simulink model "ConfiguredVirtualVehicleModel"  (R2023b)
settings: configuration reference "VehicleVariable" (kept outside this file)
StartFcn:
  | %tic
StopFcn:
  | %toc
model workspace (MAT data in the model file):
  ExtDrvCmdsSwitch : Simulink.Parameter (value not decoded)
  ExtDrvRefSwitch : Simulink.Parameter (value not decoded)
  ExtEnvSwitch : Simulink.Parameter (value not decoded)
  ExtGndSwitch : Simulink.Parameter (value not decoded)
values from neighbouring files (symbols this model uses):
  L = 2.79    [EVFmincon_custom.m]
symbols that are objects in the model workspace (value not decoded): ExtDrvCmdsSwitch, ExtDrvRefSwitch, ExtEnvSwitch, ExtGndSwitch
undefined symbols (not defined in the file or in its folder): AccelCmd, AmbTemp, BaroPress, CtrlTcuInitGear, CtrlVcuCltch1InitCmd, CurvGradRef, CurvRef, DCM, DecelCmd, Disabled, DriverAeroRes, DriverDrivelineRes, DriverInitialGear, DriverPreviewDist, DriverRollRes, DriverShiftTime, DriverTimeConst, DriverTractiveForce, EnvAbsPrs, EnvAirTemp, EnvGrvty, EnvNomFrictionScaling, EnvNominalGrade, EnvWindVelX, EnvWindVelY, EnvWindVelZ, FTP75, Gnd, Grade, HazzardCmd, HighBeamCmd, lambda_mux, LeftSignalCmd, LngRef, LowBeamCmd, LtrRef, PhiRef, PlntVehDstCGFrntAxl, PlntVehDstCGRearAxl, PlntVehInitLatPos, PlntVehInitLongPos, PlntVehInitPitchAng, PlntVehInitRollAng, PlntVehInitVertPos, PlntVehInitYawAng, PlntVehMass, PlntVehTrckWdth, PlntVehYawMomentInertia, PlntWhlLdRadius, RightSignalCmd, ScnCRMaxLatAccel, ScnCRRadius, ScnDLCGateLongPos, ScnDLCLatRef, ScnDLCLatRefOffset, ScnDLCLongRefBpt, ScnDLCLongRefStartPos, ScnDLCVehicleWidth, ScnFHCounterDwellTime, ScnFHInitialDwellTime ... (+22)
libraries: simulink x27, autolibutils x8, vehdynlibscenariocommon x7, vehdynlibviscommon x3, vehdynlibdriver x2, sim3dgroundtruthsensorlib x2, autolibshared x2, vrlib x1, autolibsharedcommon x1, sharedtransform x1, sim3dlib x1, sim3dautolib x1
(part 5 of 6)

== system ConfiguredVirtualVehicleModel/Driver Commands/Driver Commands/Longitudinal Driver/Hill Hold & Stop/Hill Hold ==
  <EngSpdOut> : Inport
  <xdot> : Inport  Port=2
  <BattSoc> : Inport  Port=3
  LngRef : Inport  Port=4
  <Grade> : Inport  Port=5
  Abs : Abs  ZeroCross=off  SaturateOnIntegerOverflow=off
  Abs1 : Abs  ZeroCross=off  SaturateOnIntegerOverflow=off
  Compare To Constant : simulink/Logic and Bit Operations/Compare To Constant  relop=<=  const=.1  OutDataTypeStr=boolean  ZeroCross=off
  Compare To Constant1 : simulink/Logic and Bit Operations/Compare To Constant  relop=>=  const=.1  OutDataTypeStr=boolean  ZeroCross=off
  Compare To Constant2 : simulink/Logic and Bit Operations/Compare To Constant  relop=<=  const=500  OutDataTypeStr=boolean  ZeroCross=off
  Compare To Constant3 : simulink/Logic and Bit Operations/Compare To Constant  relop=<=  const=5  OutDataTypeStr=boolean  ZeroCross=off
  Compare To Constant4 : simulink/Logic and Bit Operations/Compare To Constant  relop=<=  const=.1  OutDataTypeStr=boolean  ZeroCross=off
  Data Type Conversion1 : DataTypeConversion  SaturateOnIntegerOverflow=off  RndMeth=Floor
  Logical Operator : Logic  AllPortsSameDT=off  OutDataTypeStr=boolean
  Logical Operator1 : Logic  Inputs=3  AllPortsSameDT=off  OutDataTypeStr=boolean
  Logical Operator2 : Logic  Operator=OR  AllPortsSameDT=off  OutDataTypeStr=boolean
  Signal Specification : SignalSpecification  Unit=m/s
  Unit Conversion : UnitConversion
  DecelOvr : Outport
  EnblDecelOvr : Outport  Port=2
  wires:
  Compare To Constant/1 -> Logical Operator/1
  Unit Conversion/1 -> Signal Specification/1
  Logical Operator2/1 -> DecelOvr/1, Data Type Conversion1/1
  Abs1/1 -> Compare To Constant1/1
  LngRef/1 -> Abs/1
  Compare To Constant1/1 -> Logical Operator/2
  Compare To Constant3/1 -> Logical Operator1/2
  Logical Operator/1 -> Logical Operator2/2
  Compare To Constant2/1 -> Logical Operator1/1
  Data Type Conversion1/1 -> EnblDecelOvr/1
  Logical Operator1/1 -> Logical Operator2/1
  Abs/1 -> Compare To Constant/1
  Signal Specification/1 -> Compare To Constant3/1
  <EngSpdOut>/1 -> Compare To Constant2/1
  Compare To Constant4/1 -> Logical Operator1/3
  <Grade>/1 -> Abs1/1
  <xdot>/1 -> Unit Conversion/1
  <BattSoc>/1 -> Compare To Constant4/1

== system ConfiguredVirtualVehicleModel/Driver Commands/Driver Commands/Longitudinal Driver/Hill Hold & Stop/Stop Detection ==
  LngRef : Inport
  <xdot> : Inport  Port=2
  Abs2 : Abs  ZeroCross=off  SaturateOnIntegerOverflow=off
  Compare To Constant5 : simulink/Logic and Bit Operations/Compare To Constant  relop=<=  const=.1  OutDataTypeStr=boolean  ZeroCross=off
  Compare To Constant6 : simulink/Logic and Bit Operations/Compare To Constant  relop===  const=0  OutDataTypeStr=boolean  ZeroCross=off
  Cont LPF : autolibutils/Cont LPF  wc=2*pi*40  AbsoluteTolerance=auto  aMode=6
  Data Type Conversion2 : DataTypeConversion  SaturateOnIntegerOverflow=off  RndMeth=Floor
  Gain : Gain  Gain=.1
  LatchSwitchCont : autolibutils/LatchSwitchCont  aMode=6
  Logical Operator1 : Logic  Operator=NOT  AllPortsSameDT=off  OutDataTypeStr=boolean
  Logical Operator3 : Logic  AllPortsSameDT=off  OutDataTypeStr=boolean
  DecelOvrCmd : Outport
  EnblDecelOvr : Outport  Port=2
  wires:
  Compare To Constant5/1 -> Logical Operator3/1
  Logical Operator3/1 -> LatchSwitchCont/1
  LngRef/1 -> Compare To Constant6/1
  Abs2/1 -> Compare To Constant5/1
  LatchSwitchCont/1 -> EnblDecelOvr/1, Data Type Conversion2/1
  Data Type Conversion2/1 -> Gain/1
  Logical Operator1/1 -> LatchSwitchCont/2
  Compare To Constant6/1 -> Logical Operator1/1, Logical Operator3/2
  Gain/1 -> Cont LPF/1
  Cont LPF/1 -> DecelOvrCmd/1
  <xdot>/1 -> Abs2/1

== system ConfiguredVirtualVehicleModel/Driver Commands/Driver Commands/Longitudinal Driver/Longitudinal Driver/External Action Routing ==
  EnblAccelOvr : Inport  OutDataTypeStr=boolean  Unit=1  PortDimensions=1
  AccelOvrCmd : Inport  Port=2  OutDataTypeStr=double  Unit=1  PortDimensions=1
  AccelHld : Inport  Port=3  OutDataTypeStr=boolean  Unit=1  PortDimensions=1
  AccelZero : Inport  Port=4  OutDataTypeStr=boolean  Unit=1  PortDimensions=1
  EnblDecelOvr : Inport  Port=5  OutDataTypeStr=boolean  Unit=1  PortDimensions=1
  DecelOvrCmd : Inport  Port=6  OutDataTypeStr=double  Unit=1  PortDimensions=1
  DecelHld : Inport  Port=7  OutDataTypeStr=boolean  Unit=1  PortDimensions=1
  DecelZero : Inport  Port=8  OutDataTypeStr=boolean  Unit=1  PortDimensions=1
  Bus Creator2 : BusCreator  Inputs=8
  ExtActions : Outport
  wires:
  EnblAccelOvr/1 -> Bus Creator2/1  "EnblAccelOvr"
  AccelOvrCmd/1 -> Bus Creator2/2  "AccelOvrCmd"
  AccelHld/1 -> Bus Creator2/3  "AccelHld"
  AccelZero/1 -> Bus Creator2/4  "AccelZero"
  EnblDecelOvr/1 -> Bus Creator2/5  "EnblDecelOvr"
  DecelOvrCmd/1 -> Bus Creator2/6  "DecelOvrCmd"
  DecelHld/1 -> Bus Creator2/7  "DecelHld"
  DecelZero/1 -> Bus Creator2/8  "DecelZero"
  Bus Creator2/1 -> ExtActions/1  "ExtActions"

== system ConfiguredVirtualVehicleModel/Driver Commands/Driver Commands/Predictive Driver/Hill Hold & Stop/Hill Hold ==
  <EngSpdOut> : Inport
  <xdot> : Inport  Port=2
  <BattSoc> : Inport  Port=3
  LngRef : Inport  Port=4
  <Grade> : Inport  Port=5
  Abs : Abs  ZeroCross=off  SaturateOnIntegerOverflow=off
  Abs1 : Abs  ZeroCross=off  SaturateOnIntegerOverflow=off
  Compare To Constant : simulink/Logic and Bit Operations/Compare To Constant  relop=<=  const=.1  OutDataTypeStr=boolean  ZeroCross=off
  Compare To Constant1 : simulink/Logic and Bit Operations/Compare To Constant  relop=>=  const=.1  OutDataTypeStr=boolean  ZeroCross=off
  Compare To Constant2 : simulink/Logic and Bit Operations/Compare To Constant  relop=<=  const=500  OutDataTypeStr=boolean  ZeroCross=off
  Compare To Constant3 : simulink/Logic and Bit Operations/Compare To Constant  relop=<=  const=5  OutDataTypeStr=boolean  ZeroCross=off
  Compare To Constant4 : simulink/Logic and Bit Operations/Compare To Constant  relop=<=  const=.1  OutDataTypeStr=boolean  ZeroCross=off
  Data Type Conversion1 : DataTypeConversion  SaturateOnIntegerOverflow=off  RndMeth=Floor
  Logical Operator : Logic  AllPortsSameDT=off  OutDataTypeStr=boolean
  Logical Operator1 : Logic  Inputs=3  AllPortsSameDT=off  OutDataTypeStr=boolean
  Logical Operator2 : Logic  Operator=OR  AllPortsSameDT=off  OutDataTypeStr=boolean
  Signal Specification : SignalSpecification  Unit=m/s
  Unit Conversion : UnitConversion
  DecelOvr : Outport
  EnblDecelOvr : Outport  Port=2
  wires:
  Compare To Constant/1 -> Logical Operator/1
  Unit Conversion/1 -> Signal Specification/1
  Logical Operator2/1 -> DecelOvr/1, Data Type Conversion1/1
  Abs1/1 -> Compare To Constant1/1
  LngRef/1 -> Abs/1
  Compare To Constant1/1 -> Logical Operator/2
  Compare To Constant3/1 -> Logical Operator1/2
  Logical Operator/1 -> Logical Operator2/2
  Compare To Constant2/1 -> Logical Operator1/1
  Data Type Conversion1/1 -> EnblDecelOvr/1
  Logical Operator1/1 -> Logical Operator2/1
  Abs/1 -> Compare To Constant/1
  Signal Specification/1 -> Compare To Constant3/1
  <EngSpdOut>/1 -> Compare To Constant2/1
  Compare To Constant4/1 -> Logical Operator1/3
  <Grade>/1 -> Abs1/1
  <xdot>/1 -> Unit Conversion/1
  <BattSoc>/1 -> Compare To Constant4/1

== system ConfiguredVirtualVehicleModel/Driver Commands/Driver Commands/Predictive Driver/Hill Hold & Stop/Stop Detection ==
  LngRef : Inport
  <xdot> : Inport  Port=2
  Abs2 : Abs  ZeroCross=off  SaturateOnIntegerOverflow=off
  Compare To Constant5 : simulink/Logic and Bit Operations/Compare To Constant  relop=<=  const=.1  OutDataTypeStr=boolean  ZeroCross=off
  Compare To Constant6 : simulink/Logic and Bit Operations/Compare To Constant  relop===  const=0  OutDataTypeStr=boolean  ZeroCross=off
  Cont LPF : autolibutils/Cont LPF  wc=2*pi*40  AbsoluteTolerance=auto  aMode=6
  Data Type Conversion2 : DataTypeConversion  SaturateOnIntegerOverflow=off  RndMeth=Floor
  Gain : Gain  Gain=.1
  LatchSwitchCont : autolibutils/LatchSwitchCont  aMode=6
  Logical Operator1 : Logic  Operator=NOT  AllPortsSameDT=off  OutDataTypeStr=boolean
  Logical Operator3 : Logic  AllPortsSameDT=off  OutDataTypeStr=boolean
  DecelOvrCmd : Outport
  EnblDecelOvr : Outport  Port=2
  wires:
  Compare To Constant5/1 -> Logical Operator3/1
  Logical Operator3/1 -> LatchSwitchCont/1
  LngRef/1 -> Compare To Constant6/1
  Abs2/1 -> Compare To Constant5/1
  LatchSwitchCont/1 -> EnblDecelOvr/1, Data Type Conversion2/1
  Data Type Conversion2/1 -> Gain/1
  Logical Operator1/1 -> LatchSwitchCont/2
  Compare To Constant6/1 -> Logical Operator1/1, Logical Operator3/2
  Gain/1 -> Cont LPF/1
  Cont LPF/1 -> DecelOvrCmd/1
  <xdot>/1 -> Abs2/1

== system ConfiguredVirtualVehicleModel/Driver Commands/Driver Commands/Predictive Stanley Driver/Hill Hold & Stop/Hill Hold ==
  <EngSpdOut> : Inport
  <xdot> : Inport  Port=2
  <BattSoc> : Inport  Port=3
  LngRef : Inport  Port=4
  <Grade> : Inport  Port=5
  Abs : Abs  ZeroCross=off  SaturateOnIntegerOverflow=off
  Abs1 : Abs  ZeroCross=off  SaturateOnIntegerOverflow=off
  Compare To Constant : simulink/Logic and Bit Operations/Compare To Constant  relop=<=  const=.1  OutDataTypeStr=boolean  ZeroCross=off
  Compare To Constant1 : simulink/Logic and Bit Operations/Compare To Constant  relop=>=  const=.1  OutDataTypeStr=boolean  ZeroCross=off
  Compare To Constant2 : simulink/Logic and Bit Operations/Compare To Constant  relop=<=  const=500  OutDataTypeStr=boolean  ZeroCross=off
  Compare To Constant3 : simulink/Logic and Bit Operations/Compare To Constant  relop=<=  const=5  OutDataTypeStr=boolean  ZeroCross=off
  Compare To Constant4 : simulink/Logic and Bit Operations/Compare To Constant  relop=<=  const=.1  OutDataTypeStr=boolean  ZeroCross=off
  Data Type Conversion1 : DataTypeConversion  SaturateOnIntegerOverflow=off  RndMeth=Floor
  Logical Operator : Logic  AllPortsSameDT=off  OutDataTypeStr=boolean
  Logical Operator1 : Logic  Inputs=3  AllPortsSameDT=off  OutDataTypeStr=boolean
  Logical Operator2 : Logic  Operator=OR  AllPortsSameDT=off  OutDataTypeStr=boolean
  Signal Specification : SignalSpecification  Unit=m/s
  Unit Conversion : UnitConversion
  DecelOvr : Outport
  EnblDecelOvr : Outport  Port=2
  wires:
  Compare To Constant/1 -> Logical Operator/1
  Unit Conversion/1 -> Signal Specification/1
  Logical Operator2/1 -> DecelOvr/1, Data Type Conversion1/1
  Abs1/1 -> Compare To Constant1/1
  LngRef/1 -> Abs/1
  Compare To Constant1/1 -> Logical Operator/2
  Compare To Constant3/1 -> Logical Operator1/2
  Logical Operator/1 -> Logical Operator2/2
  Compare To Constant2/1 -> Logical Operator1/1
  Data Type Conversion1/1 -> EnblDecelOvr/1
  Logical Operator1/1 -> Logical Operator2/1
  Abs/1 -> Compare To Constant/1
  Signal Specification/1 -> Compare To Constant3/1
  <EngSpdOut>/1 -> Compare To Constant2/1
  Compare To Constant4/1 -> Logical Operator1/3
  <Grade>/1 -> Abs1/1
  <xdot>/1 -> Unit Conversion/1
  <BattSoc>/1 -> Compare To Constant4/1

== system ConfiguredVirtualVehicleModel/Driver Commands/Driver Commands/Predictive Stanley Driver/Hill Hold & Stop/Stop Detection ==
  LngRef : Inport
  <xdot> : Inport  Port=2
  Abs2 : Abs  ZeroCross=off  SaturateOnIntegerOverflow=off
  Compare To Constant5 : simulink/Logic and Bit Operations/Compare To Constant  relop=<=  const=.1  OutDataTypeStr=boolean  ZeroCross=off
  Compare To Constant6 : simulink/Logic and Bit Operations/Compare To Constant  relop===  const=0  OutDataTypeStr=boolean  ZeroCross=off
  Cont LPF : autolibutils/Cont LPF  wc=2*pi*40  AbsoluteTolerance=auto  aMode=6
  Data Type Conversion2 : DataTypeConversion  SaturateOnIntegerOverflow=off  RndMeth=Floor
  Gain : Gain  Gain=.1
  LatchSwitchCont : autolibutils/LatchSwitchCont  aMode=6
  Logical Operator1 : Logic  Operator=NOT  AllPortsSameDT=off  OutDataTypeStr=boolean
  Logical Operator3 : Logic  AllPortsSameDT=off  OutDataTypeStr=boolean
  DecelOvrCmd : Outport
  EnblDecelOvr : Outport  Port=2
  wires:
  Compare To Constant5/1 -> Logical Operator3/1
  Logical Operator3/1 -> LatchSwitchCont/1
  LngRef/1 -> Compare To Constant6/1
  Abs2/1 -> Compare To Constant5/1
  LatchSwitchCont/1 -> EnblDecelOvr/1, Data Type Conversion2/1
  Data Type Conversion2/1 -> Gain/1
  Logical Operator1/1 -> LatchSwitchCont/2
  Compare To Constant6/1 -> Logical Operator1/1, Logical Operator3/2
  Gain/1 -> Cont LPF/1
  Cont LPF/1 -> DecelOvrCmd/1
  <xdot>/1 -> Abs2/1

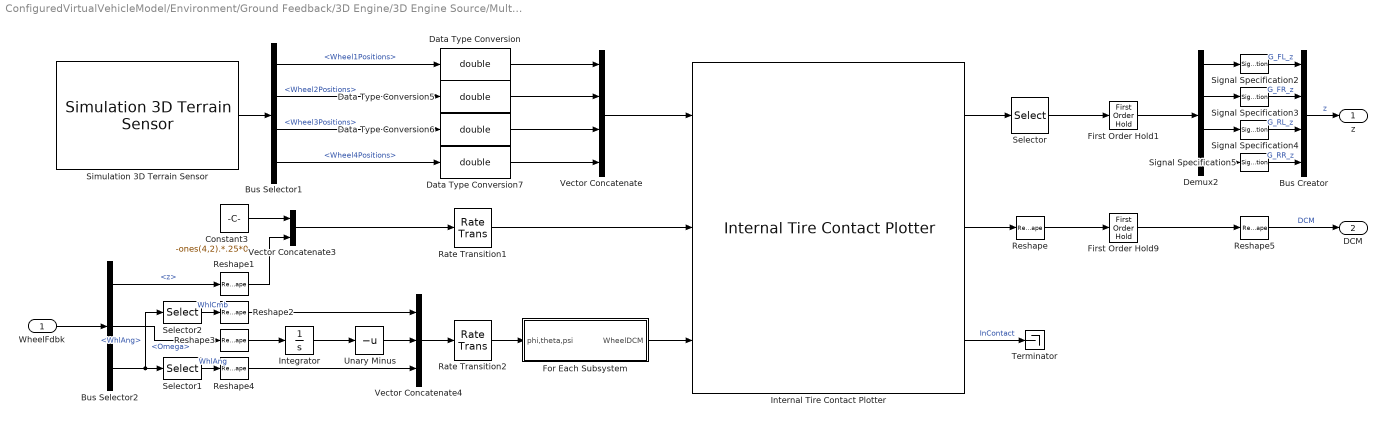
== system ConfiguredVirtualVehicleModel/Environment/Ground Feedback/3D Engine/3D Engine Source/Multiple Points ==
  WheelFdbk : Inport
  Bus Creator : BusCreator  Inputs=4
  Bus Selector1 : BusSelector  OutputSignals=Wheel1Positions,Wheel2Positions,Wheel3Positions,Wheel4Positions
  Bus Selector2 : BusSelector  OutputSignals=z,Omega,WhlAng
  Constant3 : Constant  Value=-ones(4,2).*.25*0
  Data Type Conversion{,5..7} (4 alike) : DataTypeConversion  OutDataTypeStr=double  SaturateOnIntegerOverflow=off  RndMeth=Floor
  Demux2 : Demux
  First Order Hold1 : FirstOrderHold  OutputAlgorithm=Fast (Minimize Error)  ErrorTolerance=.001
  First Order Hold9 : FirstOrderHold  InitialOutput=reshape(repmat(eye(3),1,1,4),[],1)  OutputAlgorithm=Fast (Minimize Error)  ErrorTolerance=.001
  For Each Subsystem : Subsystem  TreatAsAtomicUnit=on
  Integrator : Integrator  WrapState=on  ZeroCross=off
  Internal Tire Contact Plotter : vehdynlibviscommon/Internal Tire Contact Plotter  dispFig=off  numAxles=2  numWheelsPerAxle=2  wheelRad=.33  wheelWidth=.235  rayOrigins=[0.5 -0.5 0;0.4 -0.5 0;0.3 -0.5 0;0.19999999999999996 -0.5 0;0.099999999999999978 -0.5 0;0 -0.5 0;-0.099999999999999978 -0.5 0;-0.19999999999999996 -0.5 0;-0.3 -0.5 0;-0.4 -0.5 0;-0.5 -0.5 0;0.5 -0.4 0;0.4 -0.4 0;0.3 -0.4 0;0.19999999999999996 -0.4 0;0.099999999999999978 -0.4 0;0 -0.4 0;-0.099999999999999978 -0.4 0;-0.19999999999999996 -0.4 0;-0.3 -0.4 0;-0.4 -0.4 0;-0.5 -0.4 0;0.5 -0.3 0;0.4 -0.3 0;0.3 -0.3 0;0.19999999999999996 -0.3 0;0.099999999999999978 -0.3 0;0 -0.3 0;-0.099999999999999978 -0.3 0;-0.19999999999999996 -0.3 0;-0.3 -0.3 0;-0.4 -0.3 0;-0.5 -0.3 0;0.5 -0.19999999999999996 0;0.4 -0.19999999999999996 0;0.3 -0.19999999999999996 0;0.19999999999999996 -0.19999999999999996 0;0.099999999999999978 -0.19999999999999996 0;0 -0.19999999999999996 0;-0.099999999999999978 -0.19999999999999996 0;-0.19999999999999996 -0.19999999999999996 0;-0.3 -0.19999999999999996 0;-0.4 -0.19999999999999996 0;-0.5 -0.19999999999999996 0;0.5 -0.099999999999999978 0;0.4 -0.099999999999999978 0;0.3 -0.099999999999999978 0;0.19999999999999996 -0.099999999999999978 0;0.099999999999999978 -0.099999999999999978 0;0 -0.099999999999999978 0;-0.099999999999999978 -0.099999999999999978 0;-0.19999999999999996 -0.099999999999999978 0;-0.3 -0.099999999999999978 0;-0.4 -0.099999999999999978 0;-0.5 -0.099999999999999978 0;0.5 0 0;0.4 0 0;0.3 0 0;0.19999999999999996 0 0;0.099999999999999978 0 0;0 0 0;-0.099999999999999978 0 0;-0.19999999999999996 0 0;-0.3 0 0;-0.4 0 0;-0.5 0 0;0.5 0.099999999999999978 0;0.4 0.099999999999999978 0;0.3 0.099999999999999978 0;0.19999999999999996 0.099999999999999978 0;0.099999999999999978 0.099999999999999978 0;0 0.099999999999999978 0;-0.099999999999999978 0.099999999999999978 0;-0.19999999999999996 0.099999999999999978 0;-0.3 0.099999999999999978 0;-0.4 0.099999999999999978 0;-0.5 0.099999999999999978 0;0.5 0.19999999999999996 0;0.4 0.19999999999999996 0;0.3 0.19999999999999996 0;0.19999999999999996 0.19999999999999996 0;0.099999999999999978 0.19999999999999996 0;0 0.19999999999999996 0;-0.099999999999999978 0.19999999999999996 0;-0.19999999999999996 0.19999999999999996 0;-0.3 0.19999999999999996 0;-0.4 0.19999999999999996 0;-0.5 0.19999999999999996 0;0.5 0.3 0;0.4 0.3 0;0.3 0.3 0;0.19999999999999996 0.3 0;0.099999999999999978 0.3 0;0 0.3 0;-0.099999999999999978 0.3 0;-0.19999999999999996 0.3 0;-0.3 0.3 0;-0.4 0.3 0;-0.5 0.3 0;0.5 0.4 0;0.4 0.4 0;0.3 0.4 0;0.19999999999999996 0.4 0;0.099999999999999978 0.4 0;0 0.4 0;-0.099999999999999978 0.4 0;-0.19999999999999996 0.4 0;-0.3 0.4 0;-0.4 0.4 0;-0.5 0.4 0;0.5 0.5 0;0.4 0.5 0;0.3 0.5 0;0.19999999999999996 0.5 0;0.099999999999999978 0.5 0;0 0.5 0;-0.099999999999999978 0.5 0;-0.19999999999999996 0.5 0;-0.3 0.5 0;-0.4 0.5 0;-0.5 0.5 0]
  Rate Transition1 : RateTransition  Integrity=off  Deterministic=off  OutPortSampleTime=.01
  Rate Transition2 : RateTransition  Integrity=off  Deterministic=off  OutPortSampleTime=.01
  Reshape : Reshape  OutputDimensionality=Column vector (2-D)
  Reshape1 : Reshape  OutputDimensionality=Column vector (2-D)
  Reshape2 : Reshape  OutputDimensionality=Row vector (2-D)
  Reshape3 : Reshape  OutputDimensionality=Row vector (2-D)
  Reshape4 : Reshape  OutputDimensionality=Row vector (2-D)
  Reshape5 : Reshape  OutputDimensionality=Customize  OutputDimensions=[3,3,4]
  Selector : Selector  NumberOfDimensions=2  InputPortWidth=3  IndexOptions=Select all,Index vector (dialog)  Indices=[1 3],3  OutputSizes=1,1
  Selector1 : Selector  NumberOfDimensions=2  InputPortWidth=3  IndexOptions=Index vector (dialog),Select all  Indices=[3],1  OutputSizes=1,1
  Selector2 : Selector  NumberOfDimensions=2  InputPortWidth=3  IndexOptions=Index vector (dialog),Select all  Indices=[1],1  OutputSizes=1,1
  Signal Specification{2..5} (4 alike) : SignalSpecification  Unit=m
  Simulation 3D Terrain Sensor : sim3dgroundtruthsensorlib/Simulation 3D Terrain Sensor  Priority=1  vehTagList={'Scene Origin';'SimulinkVehicle1'}  sensorTag=Sim3dSensor1  sensorId=1  sensorName=Sim3dSensor1  vehTag=SimulinkVehicle1  tmountOffset=[0, 0, 0]  rmountOffset=[0,0,0,]  RayOrigins=[0.5 -0.5 0;0.4 -0.5 0;0.3 -0.5 0;0.19999999999999996 -0.5 0;0.099999999999999978 -0.5 0;0 -0.5 0;-0.099999999999999978 -0.5 0;-0.19999999999999996 -0.5 0;-0.3 -0.5 0;-0.4 -0.5 0;-0.5 -0.5 0;0.5 -0.4 0;0.4 -0.4 0;0.3 -0.4 0;0.19999999999999996 -0.4 0;0.099999999999999978 -0.4 0;0 -0.4 0;-0.099999999999999978 -0.4 0;-0.19999999999999996 -0.4 0;-0.3 -0.4 0;-0.4 -0.4 0;-0.5 -0.4 0;0.5 -0.3 0;0.4 -0.3 0;0.3 -0.3 0;0.19999999999999996 -0.3 0;0.099999999999999978 -0.3 0;0 -0.3 0;-0.099999999999999978 -0.3 0;-0.19999999999999996 -0.3 0;-0.3 -0.3 0;-0.4 -0.3 0;-0.5 -0.3 0;0.5 -0.19999999999999996 0;0.4 -0.19999999999999996 0;0.3 -0.19999999999999996 0;0.19999999999999996 -0.19999999999999996 0;0.099999999999999978 -0.19999999999999996 0;0 -0.19999999999999996 0;-0.099999999999999978 -0.19999999999999996 0;-0.19999999999999996 -0.19999999999999996 0;-0.3 -0.19999999999999996 0;-0.4 -0.19999999999999996 0;-0.5 -0.19999999999999996 0;0.5 -0.099999999999999978 0;0.4 -0.099999999999999978 0;0.3 -0.099999999999999978 0;0.19999999999999996 -0.099999999999999978 0;0.099999999999999978 -0.099999999999999978 0;0 -0.099999999999999978 0;-0.099999999999999978 -0.099999999999999978 0;-0.19999999999999996 -0.099999999999999978 0;-0.3 -0.099999999999999978 0;-0.4 -0.099999999999999978 0;-0.5 -0.099999999999999978 0;0.5 0 0;0.4 0 0;0.3 0 0;0.19999999999999996 0 0;0.099999999999999978 0 0;0 0 0;-0.099999999999999978 0 0;-0.19999999999999996 0 0;-0.3 0 0;-0.4 0 0;-0.5 0 0;0.5 0.099999999999999978 0;0.4 0.099999999999999978 0;0.3 0.099999999999999978 0;0.19999999999999996 0.099999999999999978 0;0.099999999999999978 0.099999999999999978 0;0 0.099999999999999978 0;-0.099999999999999978 0.099999999999999978 0;-0.19999999999999996 0.099999999999999978 0;-0.3 0.099999999999999978 0;-0.4 0.099999999999999978 0;-0.5 0.099999999999999978 0;0.5 0.19999999999999996 0;0.4 0.19999999999999996 0;0.3 0.19999999999999996 0;0.19999999999999996 0.19999999999999996 0;0.099999999999999978 0.19999999999999996 0;0 0.19999999999999996 0;-0.099999999999999978 0.19999999999999996 0;-0.19999999999999996 0.19999999999999996 0;-0.3 0.19999999999999996 0;-0.4 0.19999999999999996 0;-0.5 0.19999999999999996 0;0.5 0.3 0;0.4 0.3 0;0.3 0.3 0;0.19999999999999996 0.3 0;0.099999999999999978 0.3 0;0 0.3 0;-0.099999999999999978 0.3 0;-0.19999999999999996 0.3 0;-0.3 0.3 0;-0.4 0.3 0;-0.5 0.3 0;0.5 0.4 0;0.4 0.4 0;0.3 0.4 0;0.19999999999999996 0.4 0;0.099999999999999978 0.4 0;0 0.4 0;-0.099999999999999978 0.4 0;-0.19999999999999996 0.4 0;-0.3 0.4 0;-0.4 0.4 0;-0.5 0.4 0;0.5 0.5 0;0.4 0.5 0;0.3 0.5 0;0.19999999999999996 0.5 0;0.099999999999999978 0.5 0;0 0.5 0;-0.099999999999999978 0.5 0;-0.19999999999999996 0.5 0;-0.3 0.5 0;-0.4 0.5 0;-0.5 0.5 0]  RayDirections=[0 0 -1;0 0 -1;0 0 -1;0 0 -1;0 0 -1;0 0 -1;0 0 -1;0 0 -1;0 0 -1;0 0 -1;0 0 -1;0 0 -1;0 0 -1;0 0 -1;0 0 -1;0 0 -1;0 0 -1;0 0 -1;0 0 -1;0 0 -1;0 0 -1;0 0 -1;0 0 -1;0 0 -1;0 0 -1;0 0 -1;0 0 -1;0 0 -1;0 0 -1;0 0 -1;0 0 -1;0 0 -1;0 0 -1;0 0 -1;0 0 -1;0 0 -1;0 0 -1;0 0 -1;0 0 -1;0 0 -1;0 0 -1;0 0 -1;0 0 -1;0 0 -1;0 0 -1;0 0 -1;0 0 -1;0 0 -1;0 0 -1;0 0 -1;0 0 -1;0 0 -1;0 0 -1;0 0 -1;0 0 -1;0 0 -1;0 0 -1;0 0 -1;0 0 -1;0 0 -1;0 0 -1;0 0 -1;0 0 -1;0 0 -1;0 0 -1;0 0 -1;0 0 -1;0 0 -1;0 0 -1;0 0 -1;0 0 -1;0 0 -1;0 0 -1;0 0 -1;0 0 -1;0 0 -1;0 0 -1;0 0 -1;0 0 -1;0 0 -1;0 0 -1;0 0 -1;0 0 -1;0 0 -1;0 0 -1;0 0 -1;0 0 -1;0 0 -1;0 0 -1;0 0 -1;0 0 -1;0 0 -1;0 0 -1;0 0 -1;0 0 -1;0 0 -1;0 0 -1;0 0 -1;0 0 -1;0 0 -1;0 0 -1;0 0 -1;0 0 -1;0 0 -1;0 0 -1;0 0 -1;0 0 -1;0 0 -1;0 0 -1;0 0 -1;0 0 -1;0 0 -1;0 0 -1;0 0 -1;0 0 -1;0 0 -1;0 0 -1;0 0 -1;0 0 -1;0 0 -1;0 0 -1]  RayLengths=[20;20;20;20;20;20;20;20;20;20;20;20;20;20;20;20;20;20;20;20;20;20;20;20;20;20;20;20;20;20;20;20;20;20;20;20;20;20;20;20;20;20;20;20;20;20;20;20;20;20;20;20;20;20;20;20;20;20;20;20;20;20;20;20;20;20;20;20;20;20;20;20;20;20;20;20;20;20;20;20;20;20;20;20;20;20;20;20;20;20;20;20;20;20;20;20;20;20;20;20;20;20;20;20;20;20;20;20;20;20;20;20;20;20;20;20;20;20;20;20;20]  NumberOfWheels=4  VisualizeTraceLines=off  SampleTime=-1  aMode=2  ID=1
  Terminator : Terminator
  Unary Minus : UnaryMinus
  Vector Concatenate : Concatenate  NumInputs=4  Mode=Multidimensional array  ConcatenateDimension=3
  Vector Concatenate3 : Concatenate  Mode=Multidimensional array  ConcatenateDimension=2
  Vector Concatenate4 : Concatenate  NumInputs=3  Mode=Multidimensional array
  z : Outport
  DCM : Outport  Port=2
  wires:
  Data Type Conversion6/1 -> Vector Concatenate/3
  Selector/1 -> First Order Hold1/1
  Signal Specification5/1 -> Bus Creator/4  "G_RR_z"
  Bus Selector1/3 -> Data Type Conversion6/1  "<Wheel3Positions>"
  Demux2/2 -> Signal Specification3/1
  Data Type Conversion/1 -> Vector Concatenate/1
  Data Type Conversion5/1 -> Vector Concatenate/2
  Demux2/3 -> Signal Specification4/1
  Internal Tire Contact Plotter/1 -> Selector/1
  Internal Tire Contact Plotter/3 -> Terminator/1  "InContact"
  Vector Concatenate/1 -> Internal Tire Contact Plotter/1
  Data Type Conversion7/1 -> Vector Concatenate/4
  Bus Selector1/1 -> Data Type Conversion/1  "<Wheel1Positions>"
  Demux2/4 -> Signal Specification5/1
  Bus Creator/1 -> z/1  "z"
  Signal Specification2/1 -> Bus Creator/1  "G_FL_z"
  Bus Selector1/4 -> Data Type Conversion7/1  "<Wheel4Positions>"
  Signal Specification3/1 -> Bus Creator/2  "G_FR_z"
  Signal Specification4/1 -> Bus Creator/3  "G_RL_z"
  Bus Selector1/2 -> Data Type Conversion5/1  "<Wheel2Positions>"
  Demux2/1 -> Signal Specification2/1
  Simulation 3D Terrain Sensor/1 -> Bus Selector1/1
  Reshape5/1 -> DCM/1  "DCM"
  Internal Tire Contact Plotter/2 -> Reshape/1
  Integrator/1 -> Unary Minus/1
  Bus Selector2/2 -> Reshape3/1  "<Omega>"
  Vector Concatenate3/1 -> Rate Transition1/1
  For Each Subsystem/1(WheelDCM) -> Internal Tire Contact Plotter/3
  Reshape3/1 -> Integrator/1
  Vector Concatenate4/1 -> Rate Transition2/1
  Reshape4/1 -> Vector Concatenate4/3
  Rate Transition2/1 -> For Each Subsystem/1(phi,theta,psi)
  Reshape1/1 -> Vector Concatenate3/2
  WheelFdbk/1 -> Bus Selector2/1
  Bus Selector2/1 -> Reshape1/1  "<z>"
  Bus Selector2/3 -> Selector2/1, Selector1/1  "<WhlAng>"
  Constant3/1 -> Vector Concatenate3/1
  Reshape2/1 -> Vector Concatenate4/1
  Unary Minus/1 -> Vector Concatenate4/2
  Rate Transition1/1 -> Internal Tire Contact Plotter/2
  First Order Hold9/1 -> Reshape5/1
  Reshape/1 -> First Order Hold9/1
  First Order Hold1/1 -> Demux2/1
  Selector1/1 -> Reshape4/1  "WhlAng"
  Selector2/1 -> Reshape2/1  "WhlCmb"

== system ConfiguredVirtualVehicleModel/Environment/Ground Feedback/3D Engine/3D Engine Source/Single Point ==
  Bus Creator1 : BusCreator  Inputs=4
  Bus Selector2 : BusSelector  OutputSignals=Wheel1Positions,Wheel2Positions,Wheel3Positions,Wheel4Positions
  Constant2 : Constant  Value=repmat(eye(3),1,1,4)  SampleTime=-1
  Data Type Conversion{1..4} (4 alike) : DataTypeConversion  SaturateOnIntegerOverflow=off  RndMeth=Floor
  First Order Hold{5..8} (4 alike) : FirstOrderHold  ErrorTolerance=1
  Range Limiter{5..8} (4 alike) : Saturate  UpperLimit=1e3  LowerLimit=-1e3  ZeroCross=off
  Signal Specification{6..9} (4 alike) : SignalSpecification  Unit=m
  Simulation 3D Terrain Sensor1 : sim3dgroundtruthsensorlib/Simulation 3D Terrain Sensor  Priority=1  vehTagList={'Scene Origin';'SimulinkVehicle1'}  sensorTag=Sim3dSensor1  sensorId=1  sensorName=Sim3dSensor1  vehTag=SimulinkVehicle1  tmountOffset=[0, 0, 0]  rmountOffset=[0,0,0,]  RayOrigins=[0 0 1]  RayDirections=[0 0 -1]  RayLengths=20  NumberOfWheels=4  VisualizeTraceLines=off  SampleTime=-1  aMode=2  ID=1
  Zend Select{1..4} (4 alike) : Selector  NumberOfDimensions=2  InputPortWidth=3  IndexOptions=Select all,Index vector (dialog)  Indices=[1 3],3  OutputSizes=1,1
  z : Outport
  DCM : Outport  Port=2
  wires:
  Signal Specification6/1 -> Bus Creator1/1  "G_FL_z"
  Simulation 3D Terrain Sensor1/1 -> Bus Selector2/1
  Bus Selector2/4 -> Range Limiter8/1  "<Wheel4Positions>"
  Zend Select1/1 -> Data Type Conversion1/1
  Signal Specification7/1 -> Bus Creator1/2  "G_FR_z"
  Bus Selector2/2 -> Range Limiter6/1  "<Wheel2Positions>"
  Data Type Conversion3/1 -> First Order Hold7/1
  Data Type Conversion4/1 -> First Order Hold8/1
  Zend Select3/1 -> Data Type Conversion3/1
  First Order Hold6/1 -> Signal Specification7/1
  Zend Select2/1 -> Data Type Conversion2/1
  Data Type Conversion2/1 -> First Order Hold6/1
  Range Limiter6/1 -> Zend Select2/1
  Data Type Conversion1/1 -> First Order Hold5/1
  First Order Hold7/1 -> Signal Specification8/1
  Zend Select4/1 -> Data Type Conversion4/1
  Range Limiter8/1 -> Zend Select4/1
  Bus Selector2/1 -> Range Limiter5/1  "<Wheel1Positions>"
  First Order Hold8/1 -> Signal Specification9/1
  Bus Selector2/3 -> Range Limiter7/1  "<Wheel3Positions>"
  Range Limiter7/1 -> Zend Select3/1
  First Order Hold5/1 -> Signal Specification6/1
  Range Limiter5/1 -> Zend Select1/1
  Signal Specification8/1 -> Bus Creator1/3  "G_RL_z"
  Signal Specification9/1 -> Bus Creator1/4  "G_RR_z"
  Bus Creator1/1 -> z/1  "z"
  Constant2/1 -> DCM/1  "DCM"

== system ConfiguredVirtualVehicleModel/Environment/Subsystem/Estimated Grade/Variant Subsystem/Three-Axle ==
  Gnd : Inport
  Selector : Selector  InputPortWidth=6  IndexOptions=Index vector (dialog)  Indices=[1 2]  OutputSizes=1
  Selector1 : Selector  InputPortWidth=6  IndexOptions=Index vector (dialog)  Indices=[5 6]  OutputSizes=1
  F : Outport
  R : Outport  Port=2
  wires:
  Selector/1 -> F/1
  Gnd/1 -> Selector1/1, Selector/1
  Selector1/1 -> R/1

== system ConfiguredVirtualVehicleModel/Environment/Subsystem/Estimated Grade/Variant Subsystem/Two-Axle ==
  Gnd : Inport
  Selector : Selector  InputPortWidth=4  IndexOptions=Index vector (dialog)  Indices=[1 2]  OutputSizes=1
  Selector1 : Selector  InputPortWidth=4  IndexOptions=Index vector (dialog)  Indices=[3 4]  OutputSizes=1
  F : Outport
  R : Outport  Port=2
  wires:
  Selector1/1 -> R/1
  Selector/1 -> F/1
  Gnd/1 -> Selector1/1, Selector/1

== system ConfiguredVirtualVehicleModel/Environment/Varying Friction/Varying Friction/Road Track Friction/2D Lookup Tbl for Scaling Fctr (Lambda) ==
  XWhl : Inport  Partition=on  PartitionDimension=1  PartitionWidth=1  PartitionOffset=0
  YWhl : Inport  Port=2  Partition=on  PartitionDimension=1  PartitionWidth=1  PartitionOffset=0
  XBpt : Inport  Port=3
  YBpt : Inport  Port=4
  2-D Lookup Table : Lookup_n-D  BreakpointsForDimension1Source=Input port  BreakpointsForDimension1=xbr  BreakpointsForDimension2Source=Input port  BreakpointsForDimension2=ybr  Table=mutable  ExtrapMethod=Clip  InternalRulePriority=Speed  RndMeth=Simplest
      settings: InputPortMap=u0,u1,p5,p7
  For Each : ForEach  DisableCoverage=on
  Lambda for each whl : Outport  ConcatenationDimension=1
  wires:
  XWhl/1 -> 2-D Lookup Table/1
  YWhl/1 -> 2-D Lookup Table/2
  2-D Lookup Table/1 -> Lambda for each whl/1
  XBpt/1 -> 2-D Lookup Table/3
  YBpt/1 -> 2-D Lookup Table/4

== system ConfiguredVirtualVehicleModel/Environment/Varying Friction/Varying Friction/Road Track Friction/Creating Inertial Frm Bpt ==
  XCg : Inport
  YCg : Inport  Port=2
  Enable : EnablePort
  Add : Sum
  Add1 : Sum
  Constant1 : Constant  Value=ybr
  Constant3 : Constant  Value=xbr
  XBpt : Outport
  YBpt : Outport  Port=2
  wires:
  Add/1 -> XBpt/1
  Constant1/1 -> Add1/1
  Add1/1 -> YBpt/1
  Constant3/1 -> Add/2
  YCg/1 -> Add1/2
  XCg/1 -> Add/1

== system ConfiguredVirtualVehicleModel/Environment/Varying Friction/Varying Friction/Road Track Friction/En at t = 0 ==
  Clock1 : Clock
  Compare To Zero : simulink/Logic and Bit Operations/Compare To Zero  relop===  OutDataTypeStr=boolean
  Constant : Constant
  Constant2 : Constant  Value=0
  Switch1 : Switch  Criteria=u2 > Threshold  SaturateOnIntegerOverflow=off  InputSameDT=off
  Out1 : Outport
  wires:
  Clock1/1 -> Compare To Zero/1
  Constant2/1 -> Switch1/3
  Constant/1 -> Switch1/1
  Switch1/1 -> Out1/1
  Compare To Zero/1 -> Switch1/2

== system ConfiguredVirtualVehicleModel/Scenarios/Reference Generator/Reference Generator/3D Engine/3D Engine ==
  VehFdbk : Inport
  Bus Selector : BusSelector  OutputSignals=Body.InertFrm.Geom.Disp.X,Body.InertFrm.Geom.Disp.Y,Body.InertFrm.Geom.Disp.Z,Body.InertFrm.Cg.Ang.phi,Body.InertFrm.Cg.Ang.theta,Body.InertFrm.Cg.Ang.psi
  Bus Selector1 : BusSelector  OutputSignals=Driver.LightsFdbk.HighBeamFdbk,Driver.LightsFdbk.LowBeamFdbk,Driver.LightsFdbk.BrakeLightFdbk,Driver.LightsFdbk.ReverseLightFdbk,Driver.LightsFdbk.LeftSignalFdbk,Driver.LightsFdbk.RightSignalFdbk  OutputAsBus=on
  Bus Selector2 : BusSelector  OutputSignals=Suspension.SuspWheel.dz,Wheels.Wheels.Omega,Suspension.SuspWheel.WhlAng
  Bus to Vector : BusToVector
  Constant2 : Constant  Value=0  OutDataTypeStr=single
  Data Type Conversion{1..2,4..10,12} (10 alike) : DataTypeConversion  OutDataTypeStr=single  SaturateOnIntegerOverflow=off  RndMeth=Floor
  Demux{,1..3} (4 alike) : Demux
  Integrator : Integrator  WrapState=on  WrappedStateUpperValue=2*pi  WrappedStateLowerValue=0  ZeroCross=off
  Part Rotation Concatenation : Subsystem
  Part Translation Concatenation : Subsystem
  Rate Transition : RateTransition  OutPortSampleTime=dt3D
  Scale : Subsystem
  Selector : Selector  NumberOfDimensions=2  InputPortWidth=3  IndexOptions=Index vector (dialog),Select all  Indices=[3],1  OutputSizes=1,1
  Selector1 : Selector  NumberOfDimensions=2  InputPortWidth=3  IndexOptions=Index vector (dialog),Select all  Indices=[1],1  OutputSizes=1,1
  Simulation 3D Scene Configuration : sim3dlib/Simulation 3D Scene Configuration  Priority=0  ProjectFormat=Default Scenes  SceneDesc=Open surface  ProjectName=/usr/local/MATLAB/R2023b/toolbox/shared/sim3d_projects/automotive_project_linux/UE/LinuxNoEditor/AutoVrtlEnv.sh  ScenePath=/Game/Maps/HwStrght  EnableOpenDRIVE=off  vehTagList={'Custom';'Scene Origin';'SimulinkVehicle1'}  vehTag=SimulinkVehicle1  FreeCameraInitialTranslation=[0, 0, 0]  FreeCameraDefaultInitialTranslation=[-6, 0, 2]  FreeCameraInitialRotation=[0, 0, 0]  FreeCameraDefaultInitialRotation=[0, -15, 0]  OpVisEn=off  Ts=dt3D  EnableWindow=on  EnableRemoteAccess=off  EnableWeather=off  SunAltitude=40.0  SunAzimuth=90  clouds=10  wind=1  fog=0  rain=0  EnableGeospatial=off  OriginHeight=200  OriginLatitude=40.744652  OriginLongitude=-73.988864  MapStyle=Aerial  AdditionalAssetIDs=[]  UseAdvancedSunSky=off  SolarTime=11  TimeZone=-5  Day=21  Month=9  Year=2022  UseDaylightSavingTime=on  DSTStartDay=10  DSTStartMonth=3  DSTEndDay=3  DSTEndMonth=11  DSTSwitchHour=2  sensorTag=MainCamera2  sensorId=2  sensorName=MainCamera2  mountLoc=Origin  offsetFlag=off  tmountOffset=[0, 0, 0]  rmountOffset=[0, 0, 0]  HorizontalResolution=1280  VerticalResolution=720  HorizontalFOV=60  mountPoint=[0 0 0]  mountOrientation=[0 0 0]  aMode=2  ID=2  GeoTrigger=Inactive
      settings: LibrarySourceBlock=vdynlib/Vehicle Scenarios/Sim3D/Sim3D Core/Simulation 3D Scene Configuration
  Simulation 3D Vehicle : sim3dautolib/Simulation 3D Vehicle  Priority=-1  PassVehMesh=Muscle car  MeshPath=/MathWorksSimulation/Vehicles/Muscle/Meshes/SK_MuscleCar.SK_MuscleCar  VehColor=Red  ActorName=SimulinkVehicle1  VehLightsControl=on  HeadlightColor=[ 1, 1, 1 ]  HighBeamIntensity=100000  LowBeamIntensity=60000  HighBeamConeAngle=1.22  LowBeamConeAngle=1.22  LeftHeadlightOrientation=[ 0, 0 ]  RightHeadlightOrientation=[ 0, 0 ]  BrakelightIntensity=500  ReverselightIntensity=500  SignallightIntensity=500  SignallightPeriod=1  SignalPulseWidth=50  Translation=[PlntVehInitLongPos PlntVehInitLatPos -PlntVehInitVertPos; 0 0 0; 0 0 0; 0 0 0; 0 0 0]  Rotation=[PlntVehInitRollAng PlntVehInitPitchAng PlntVehInitYawAng; 0 0 0; 0 0 0; 0 0 0; 0 0 0]  Scale=ones( 5, 3 )  SampleTime=dt3D  ActorType=SimulinkVehicle  ID=1  aMode=2  ActorTag=SimulinkVehicle1
  Unary Minus : UnaryMinus
  Unary Minus1 : UnaryMinus
  wires:
  Unary Minus/1 -> Demux/1
  Unary Minus1/1 -> Demux3/1
  Selector1/1 -> Data Type Conversion2/1
  Selector/1 -> Data Type Conversion9/1
  Bus Selector1/1 -> Bus to Vector/1
  Bus Selector/3 -> Data Type Conversion6/1  "<Z>"
  Bus Selector/5 -> Data Type Conversion8/1  "<theta>"
  Bus Selector/6 -> Data Type Conversion10/1  "<psi>"
  Bus Selector/2 -> Data Type Conversion5/1  "<Y>"
  Bus Selector/1 -> Data Type Conversion4/1  "<X>"
  Data Type Conversion7/1 -> Part Rotation Concatenation/1(Body Roll)
  Data Type Conversion4/1 -> Part Translation Concatenation/1(BodyX)
  Constant2/1 -> Part Translation Concatenation/4(WheelFrontLeftX), Part Translation Concatenation/11(WheelRearRightY), Part Translation Concatenation/10(WheelRearLeftY), Part Translation Concatenation/9(WheelFrontRightY), Part Translation Concatenation/8(WheelFrontLeftY), Part Translation Concatenation/7(WheelRearRightX), Part Translation Concatenation/6(WheelRearLeftX), Part Translation Concatenation/5(WheelFrontRightX)
  Data Type Conversion10/1 -> Part Rotation Concatenation/3(Body Yaw)
  Data Type Conversion5/1 -> Part Translation Concatenation/2(BodyY)
  Data Type Conversion8/1 -> Part Rotation Concatenation/2(Body Ptich)
  Data Type Conversion1/1 -> Unary Minus/1
  Integrator/1 -> Data Type Conversion1/1
  Demux1/2 -> Part Rotation Concatenation/13(WheelFrontRight Yaw)
  Demux1/1 -> Part Rotation Concatenation/12(WheelFrontLeft Yaw)
  Data Type Conversion9/1 -> Demux1/1
  Bus Selector2/2 -> Integrator/1  "<Omega>"
  Bus Selector2/3 -> Selector1/1, Selector/1  "<WhlAng>"
  Demux2/4 -> Part Rotation Concatenation/11(WheelRearRight Roll)
  Demux2/3 -> Part Rotation Concatenation/10(WheelRearLeft Roll)
  Demux2/2 -> Part Rotation Concatenation/9(WheelFrontRight Roll)
  Demux2/1 -> Part Rotation Concatenation/8(WheelFrontLeft Roll)
  Demux1/3 -> Part Rotation Concatenation/14(WheelRearLeft Yaw)
  Demux1/4 -> Part Rotation Concatenation/15(WheelRearRight Yaw)
  Data Type Conversion6/1 -> Part Translation Concatenation/3(BodyZ)
  VehFdbk/1 -> Rate Transition/1
  Demux3/2 -> Part Translation Concatenation/13(WheelFrontRightZ)
  Demux3/1 -> Part Translation Concatenation/12(WheelFrontLeftZ)
  Demux3/3 -> Part Translation Concatenation/14(WheelRearLeftZ)
  Demux3/4 -> Part Translation Concatenation/15(WheelRearRightZ)
  Data Type Conversion12/1 -> Unary Minus1/1
  Part Translation Concatenation/1(ConcatOut) -> Simulation 3D Vehicle/1
  Part Rotation Concatenation/1(ConcatOut) -> Simulation 3D Vehicle/2
  Bus Selector/4 -> Data Type Conversion7/1  "<phi>"
  Data Type Conversion2/1 -> Demux2/1
  Demux/1 -> Part Rotation Concatenation/4(WheelFrontLeft Pitch)
  Demux/2 -> Part Rotation Concatenation/5(WheelFrontRight Pitch)
  Demux/3 -> Part Rotation Concatenation/6(WheelRearLeft Pitch)
  Demux/4 -> Part Rotation Concatenation/7(WheelRearRight Ptich)
  Scale/1(ScaleOut) -> Simulation 3D Vehicle/3
  Rate Transition/1 -> Bus Selector1/1, Bus Selector2/1, Bus Selector/1
  Bus Selector2/1 -> Data Type Conversion12/1  "<dz>"
  Bus to Vector/1 -> Simulation 3D Vehicle/4

== system ConfiguredVirtualVehicleModel/Scenarios/Reference Generator/Reference Generator/3D Engine/3D Engine Disabled ==
  VehFdbk : Inport
  Terminator : Terminator
  wires:
  VehFdbk/1 -> Terminator/1

== system ConfiguredVirtualVehicleModel/Scenarios/Reference Generator/Reference Generator/Reference Generator/Braking ==
  "VehFdbk " : Inport
  Bus Creator : BusCreator  Inputs=3
  Bus Creator1 : BusCreator  Inputs=14
  Constant{,2..3,8} (4 alike) : Constant  Value=0
  Constant{1,4..7,9..12} (9 alike) : Constant  Value=false
  Ground : Ground
  Ground1 : Ground
  Ground2 : Ground
  Signal Specification : SignalSpecification  Unit=rad
  Signal Specification1 : SignalSpecification  Unit=one
  Signal Specification2 : SignalSpecification  Unit=one
  Straight Maneuver Reference Generator : vehdynlibscenariocommon/Straight Maneuver Reference Generator  t_start=t_start  ax=ax  xdot_r=xdot_r  xdotUnit=mph  brakingParam=Longitudinal displacement  t_brake=t_brake  x_brake=x_brake  ax_dec=ax_dec  BufferSize=40960  fixhw=on  faultTracking=on  xdot_rmax=1  xdot_rmean=2  r_max=1  hw_max=3  SimStopOnFault=off  aMode=2
  " Vis" : Outport
  " Ref" : Outport  Port=2
  " Fdbk" : Outport  Port=3
  wires:
  Straight Maneuver Reference Generator/1 -> Bus Creator1/1  "XRef"
  Ground/1 -> Bus Creator/1  "XRef"
  Ground2/1 -> Bus Creator/3  "ZRef"
  Constant6/1 -> Bus Creator1/7  "EnblAccelOvr"
  Constant/1 -> Bus Creator1/2  "LtrlRef"
  Bus Creator1/1 -> " Ref"/1
  Constant5/1 -> Bus Creator1/6  "SteerZero"
  Constant3/1 -> Signal Specification/1
  Constant7/1 -> Bus Creator1/9  "AccelHld"
  Signal Specification1/1 -> Bus Creator1/8  "AccelOvrCmd"
  Ground1/1 -> Bus Creator/2  "YRef"
  Signal Specification/1 -> Bus Creator1/4  "SteerOvrCmd"
  Bus Creator/1 -> " Vis"/1
  Constant12/1 -> Bus Creator1/14  "DecelZero"
  Constant1/1 -> Bus Creator1/3  "EnblSteerCmd"
  Constant10/1 -> Bus Creator1/11  "EnblDecelCmd"
  Constant11/1 -> Bus Creator1/13  "DecelHld"
  Signal Specification2/1 -> Bus Creator1/12  "DecelOvrCmd"
  Constant2/1 -> Signal Specification2/1
  Constant8/1 -> Signal Specification1/1
  Constant4/1 -> Bus Creator1/5  "SteerHld"
  Constant9/1 -> Bus Creator1/10  "AccelZero"
  "VehFdbk "/1 -> Straight Maneuver Reference Generator/1, " Fdbk"/1

== system ConfiguredVirtualVehicleModel/Scenarios/Reference Generator/Reference Generator/Reference Generator/Constant Radius ==
  VehFdbk : Inport
  Constant Radius : vehdynlibscenariocommon/Constant Radius  VariantControl=manType ==5  t_start=t_start  xdot_r=xdot_r  xdotUnit=mph  R=R  X_o=X_o  Y_o=Y_o  psi_o=psi_o  vehW=6  ay_max=cr_ay_max  steerDir=off  ay_stop=off  use3DCones=off  aMode=2
  " Vis" : Outport
  " Ref" : Outport  Port=2
  " Fdbk" : Outport  Port=3
  wires:
  VehFdbk/1 -> Constant Radius/1
  Constant Radius/2 -> " Ref"/1
  Constant Radius/3 -> " Fdbk"/1
  Constant Radius/1 -> " Vis"/1

== system ConfiguredVirtualVehicleModel/Scenarios/Reference Generator/Reference Generator/Reference Generator/Double Lane Change ==
  "VehFdbk " : Inport
  Double Lane Change : vehdynlibscenariocommon/Lane Change Reference Generator  VariantControl=Variant1  ssMode=Initialize from model  ssVar=dlcSS35mph  t_start=t_start  XGate=XGate  xdot_r=xdot_r  xdotUnit=mph  xStart=xStart  vehW=vehW  latoff=latoff  lattoff=VEH.InitialLatPosition  centerSwitch=on  xSimStop=off  ssDefault=off  latRefbp=latRefbp  latRef=latRef  X_o=X_o  Y_o=Y_o  psi_o=phi_o  ssTol=1e-3  ssMaxTime=30  ssWSName=dlcSS35mph  aMode=2  use3DCones=off
      link override ISO 3888-2/Lateral Reference: LabelModeActiveChoice=1
  " Vis" : Outport  VectorParamsAs1DForOutWhenUnconnected=off
  " Ref" : Outport  Port=2  VectorParamsAs1DForOutWhenUnconnected=off
  " Fdbk" : Outport  Port=3  VectorParamsAs1DForOutWhenUnconnected=off
  wires:
  "VehFdbk "/1 -> " Fdbk"/1, Double Lane Change/1
  Double Lane Change/1 -> " Vis"/1
  Double Lane Change/2 -> " Ref"/1

== system ConfiguredVirtualVehicleModel/Scenarios/Reference Generator/Reference Generator/Reference Generator/Drive Cycle ==
  "VehFdbk " : Inport
  Bus Creator : BusCreator  Inputs=3
  Bus Creator1 : BusCreator  Inputs=16
  Bus Selector : BusSelector  OutputSignals=Body.InertFrm.Cg.Disp.X
  Constant{,2..3,8,13..15,17} (8 alike) : Constant  Value=0
  Constant{1,4..7,9..12} (9 alike) : Constant  Value=false
  Constant16 : Constant  Value=[0 0]
  Drive Cycle Source : autolibshared/Drive Cycle Source  cycleVar=FTP75  fileVar=L:\Bauto\matlab\test\toolbox\shared\autoblks\scenario\adac.txt  tfinal="2474  seconds"  cycleRepeat=off  outAccPort=off  outGearPort=off  gearList=No gear data  t_wot1=t_start  xdot_woto=0  xdot_wot1=xdot_r  t_wot2=t_wot2  xdot_wot2=0  t_wotend=ScnSimTime  srcUnit=m/s  outUnit=mph  srcAccUnit=m/s/s  outAccUnit=m/s^2  dt=0  aMode=6  faultOption=off  velBnd=2  velBndUnit=mph  inUnit=m/s  timeBnd=1  failOption=off  stopSim=off  maxFaultCnt=10  maxFaultTime=2  maxTotFaultTime=15  traceOption=off  dtTrace=1  traceWindow=10  lastDCname=FTP75  lastOutUnit=mph  lastDT=0  lastTB=1  lastSB=2  forceCalcBound=off
  Mux : Mux  Inputs=2
  Signal Specification : SignalSpecification  Unit=rad
  Signal Specification1 : SignalSpecification  Unit=one
  Signal Specification2 : SignalSpecification  Unit=one
  " Vis" : Outport  VectorParamsAs1DForOutWhenUnconnected=off
  " Ref" : Outport  Port=2  VectorParamsAs1DForOutWhenUnconnected=off
  " Fdbk" : Outport  Port=3  VectorParamsAs1DForOutWhenUnconnected=off
  wires:
  Constant17/1 -> Bus Creator1/4  "CurvRef"
  Constant13/1 -> Bus Creator/1  "XRef"
  Constant14/1 -> Bus Creator/2  "YRef"
  Constant15/1 -> Bus Creator/3  "ZRef"
  Bus Creator/1 -> " Vis"/1
  Bus Creator1/1 -> " Ref"/1
  Constant/1 -> Bus Creator1/2  "LtrlRef"
  Constant1/1 -> Bus Creator1/5  "EnblSteerCmd"
  Constant3/1 -> Signal Specification/1
  Signal Specification/1 -> Bus Creator1/6  "SteerOvrCmd"
  Constant5/1 -> Bus Creator1/8  "SteerZero"
  Constant10/1 -> Bus Creator1/13  "EnblDecelCmd"
  Constant11/1 -> Bus Creator1/15  "DecelHld"
  Signal Specification1/1 -> Bus Creator1/10  "AccelOvrCmd"
  Constant9/1 -> Bus Creator1/12  "AccelZero"
  Constant7/1 -> Bus Creator1/11  "AccelHld"
  Constant6/1 -> Bus Creator1/9  "EnblAccelOvr"
  Constant12/1 -> Bus Creator1/16  "DecelZero"
  Signal Specification2/1 -> Bus Creator1/14  "DecelOvrCmd"
  Constant4/1 -> Bus Creator1/7  "SteerHld"
  Constant8/1 -> Signal Specification1/1
  Constant2/1 -> Signal Specification2/1
  Drive Cycle Source/1 -> Bus Creator1/1  "LngRef"
  Constant16/1 -> Mux/2  "LtrlRef"
  Mux/1 -> Bus Creator1/3  "PoseRef"
  Bus Selector/1 -> Mux/1  "<X>"
  "VehFdbk "/1 -> Bus Selector/1, " Fdbk"/1

== system ConfiguredVirtualVehicleModel/Scenarios/Reference Generator/Reference Generator/Reference Generator/Fishhook ==
  "VehFdbk " : Inport
  Bus Creator : BusCreator  Inputs=3
  Constant : Constant  Value=0
  Constant1 : Constant  Value=0
  Constant2 : Constant  Value=0
  Fishhook : vehdynlibscenariocommon/Fishhook  ssMode=Initialize from model  ssVar=fh50mph  t_start=t_start  xdot_r=xdot_r  xdotUnit=mph  steerRate=steerRate  steerA=steerAFH  pFdbk=off  tDwell1=tDwell1  tDwell2=tDwell2  tSteer3=tSteer3  pZero=pZero  steerDir=off  ssDefault=off  X_o=X_o  Y_o=Y_o  psi_o=psi_o  ssTol=1  ssMaxTime=30  ssWSName=fh50mph  aMode=2
  " Vis" : Outport  VectorParamsAs1DForOutWhenUnconnected=off
  " Ref" : Outport  Port=2  VectorParamsAs1DForOutWhenUnconnected=off
  " Fdbk" : Outport  Port=3  VectorParamsAs1DForOutWhenUnconnected=off
  wires:
  Constant/1 -> Bus Creator/1  "XRef"
  Constant1/1 -> Bus Creator/2  "YRef"
  Constant2/1 -> Bus Creator/3  "ZRef"
  Bus Creator/1 -> " Vis"/1
  Fishhook/1 -> " Ref"/1
  "VehFdbk "/1 -> " Fdbk"/1, Fishhook/1

== system ConfiguredVirtualVehicleModel/Scenarios/Reference Generator/Reference Generator/Reference Generator/Increasing Steer ==
  "VehFdbk " : Inport
  Bus Creator : BusCreator  Inputs=3
  Constant : Constant  Value=0
  Constant1 : Constant  Value=0
  Constant2 : Constant  Value=0
  Increasing Steer : vehdynlibscenariocommon/Slowly Increasing Steer  VariantControl=1  ssMode=Initialize from model  ssVar=is50mph  t_start=t_start  xdot_r=xdot_r  xdotUnit=mph  omega_hw=omega_hw  theta_max=theta_max  t_stop=t_stop  ay_max=ay_max  steerDir=off  ay_stop=on  ssDefault=off  X_o=X_o  Y_o=Y_o  psi_o=psi_o  ssTol=1  ssMaxTime=30  ssWSName=is50mph  aMode=2
  " Vis" : Outport  VectorParamsAs1DForOutWhenUnconnected=off
  " Ref" : Outport  Port=2  VectorParamsAs1DForOutWhenUnconnected=off
  " Fdbk" : Outport  Port=3  VectorParamsAs1DForOutWhenUnconnected=off
  wires:
  "VehFdbk "/1 -> " Fdbk"/1, Increasing Steer/1
  Bus Creator/1 -> " Vis"/1
  Increasing Steer/1 -> " Ref"/1  "LtrlRef"
  Constant2/1 -> Bus Creator/3  "ZRef"
  Constant1/1 -> Bus Creator/2  "YRef"
  Constant/1 -> Bus Creator/1  "XRef"

== system ConfiguredVirtualVehicleModel/Scenarios/Reference Generator/Reference Generator/Reference Generator/No Commands ==
  "VehFdbk " : Inport
  Bus Creator : BusCreator  Inputs=3
  Bus Creator1 : BusCreator  Inputs=16
  Constant{,2..3,8,13..15,17..18} (9 alike) : Constant  Value=0
  Constant{1,4..7,9..12} (9 alike) : Constant  Value=false
  Constant16 : Constant  Value=zeros(1,3)
  Signal Specification : SignalSpecification  Unit=rad
  Signal Specification1 : SignalSpecification  Unit=one
  Signal Specification2 : SignalSpecification  Unit=one
  Signal Specification3 : SignalSpecification  Unit=m/s
  Signal Specification4 : SignalSpecification  Unit=m
  Signal Specification5 : SignalSpecification  Unit=m
  Signal Specification6 : SignalSpecification  Unit=m
  " Vis" : Outport  VectorParamsAs1DForOutWhenUnconnected=off
  " Ref" : Outport  Port=2  VectorParamsAs1DForOutWhenUnconnected=off
  " Fdbk" : Outport  Port=3  VectorParamsAs1DForOutWhenUnconnected=off
  wires:
  Constant16/1 -> Bus Creator1/3  "PoseRef"
  Constant17/1 -> Bus Creator1/4  "CurvRef"
  Constant5/1 -> Bus Creator1/8  "SteerZero"
  Constant8/1 -> Signal Specification1/1
  Constant11/1 -> Bus Creator1/15  "DecelHld"
  Signal Specification1/1 -> Bus Creator1/10  "AccelOvrCmd"
  Constant/1 -> Bus Creator1/2  "LtrlRef"
  Signal Specification4/1 -> Bus Creator/1  "XRef"
  Constant6/1 -> Bus Creator1/9  "EnblAccelOvr"
  Constant7/1 -> Bus Creator1/11  "AccelHld"
  Signal Specification6/1 -> Bus Creator/3  "ZRef"
  Bus Creator/1 -> " Vis"/1
  "VehFdbk "/1 -> " Fdbk"/1
  Constant12/1 -> Bus Creator1/16  "DecelZero"
  Constant4/1 -> Bus Creator1/7  "SteerHld"
  Bus Creator1/1 -> " Ref"/1
  Signal Specification2/1 -> Bus Creator1/14  "DecelOvrCmd"
  Signal Specification3/1 -> Bus Creator1/1  "LngRef"
  Constant9/1 -> Bus Creator1/12  "AccelZero"
  Constant3/1 -> Signal Specification/1
  Constant1/1 -> Bus Creator1/5  "EnblSteerCmd"
  Signal Specification/1 -> Bus Creator1/6  "SteerOvrCmd"
  Constant10/1 -> Bus Creator1/13  "EnblDecelCmd"
  Constant2/1 -> Signal Specification2/1
  Constant18/1 -> Signal Specification3/1
  Constant13/1 -> Signal Specification4/1
  Signal Specification5/1 -> Bus Creator/2  "YRef"
  Constant14/1 -> Signal Specification5/1
  Constant15/1 -> Signal Specification6/1
